simulink model "Velocity"  (R2018a)
settings: Solver=ode113  StartTime=0.0  StopTime=10.0  RelTol=1e-3
settings Model: Creator=28718  LastModifiedBy=28718

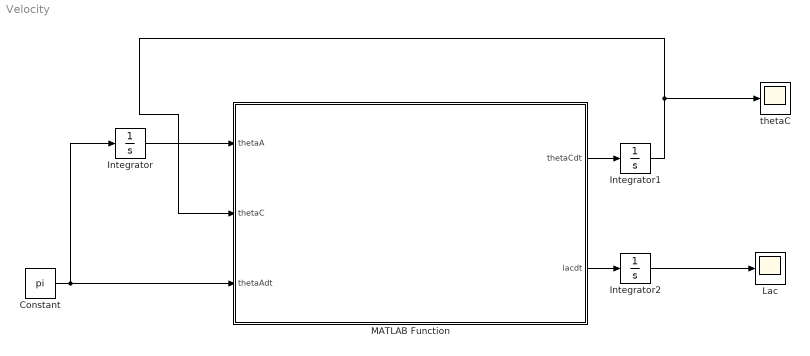
== system Velocity ==
  Constant : Constant  Value=pi
  Integrator : Integrator
  Integrator1 : Integrator
  Integrator2 : Integrator  InitialCondition=5
  Lac : Scope
  MATLAB Function : MATLAB Function  TreatAsAtomicUnit=on
  thetaC : Scope
  wires:
  Constant/1 -> Integrator/1, MATLAB Function/3(thetaAdt)
  Integrator/1 -> MATLAB Function/1(thetaA)
  MATLAB Function/1(thetaCdt) -> Integrator1/1
  Integrator1/1 -> thetaC/1, MATLAB Function/2(thetaC)
  MATLAB Function/2(lacdt) -> Integrator2/1
  Integrator2/1 -> Lac/1

== matlab function Velocity/MATLAB Function ==
  data: thetaA input; thetaCdt output; thetaC input; thetaAdt input; lacdt output
function [thetaCdt, lacdt] = fcn(thetaA, thetaC, thetaAdt)
lab=1;
lbc=4;
thetaCdt =(lab*thetaAdt*cos(thetaA))/(lbc*cos(thetaC));
lacdt =-(lab*thetaAdt*(cos(thetaA)*sin(thetaC) + cos(thetaC)*sin(thetaA)))/cos(thetaC);
end
